simulink model "lab_8_ex_2"  (R2022b)
settings: Solver=VariableStepAuto  StartTime=0.0  StopTime=10.0  RelTol=1e-3
values from neighbouring files (symbols this model uses):
  A = [-2 0 0 0 0 1 0 0 0 0 4 -3 ... (16 elements, 4x4)]    [lab_8.mat]    (also in laba9_last.m = [5 -7 -5 1)
  C = [1 -1 3 3 ... (first row only)    [laba9_last.m]
  L = inv(Q)*Y    [laba9_last.m]
settings Model: Creator=osini  LastModifiedBy=osini
settings DebuggingCC: UnconnectedInputMsg=warning  UnconnectedOutputMsg=warning  UnconnectedLineMsg=warning
settings ModelReferenceCC: EnableRefExpFcnMdlSchedulingChecks=on
settings RTWCC: DLArmComputeVersion=19.05

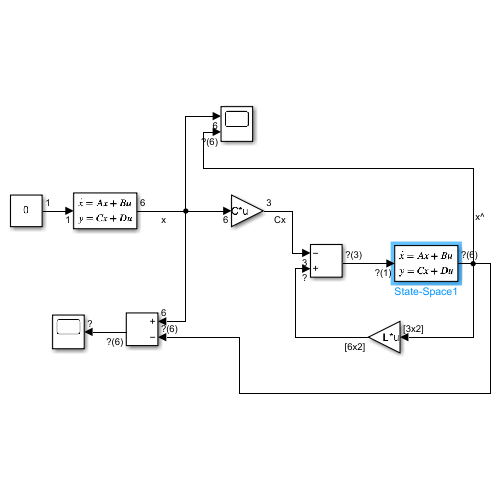
[thumbnail: Simulink's stored preview of the top-level diagram]
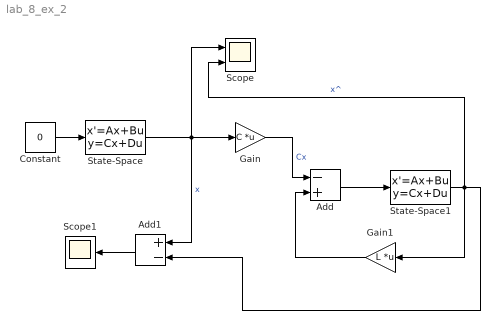
== system lab_8_ex_2 ==
  Add : Sum  Inputs=-+
  Add1 : Sum  Inputs=+-
  Constant : Constant  Value=0
  Gain : Gain  Gain=C  Multiplication=Matrix(K*u)
  Gain1 : Gain  Gain=L  Multiplication=Matrix(K*u)
  Scope : Scope  NumInputPorts=2
  Scope1 : Scope
  State-Space : StateSpace  A=A  B=[0;0;0;0;0;0]  C=eye(6,6)  D=[0;0;0;0;0;0]  InitialCondition=[1;1;1;1;1;1]
  State-Space1 : StateSpace  A=A  B=zeros(6,1)  C=eye(6)  D=zeros(6,1)  InitialCondition=[2;0;0;-1;1;1]
  wires:
  State-Space/1 -> Add1/1, Gain/1, Scope/1  "x"
  Gain/1 -> Add/1  "Cx"
  Constant/1 -> State-Space/1
  Add/1 -> State-Space1/1
  State-Space1/1 -> Add1/2, Gain1/1, Scope/2  "x^"
  Gain1/1 -> Add/2
  Add1/1 -> Scope1/1
